simulink model "SIMULADOR_ENCODER"  (R2018a)
settings: Solver=FixedStepDiscrete  StartTime=0.0  StopTime=4  FixedStep=0.001  RelTol=1e-3
libraries: simulink x1
settings Model: Creator=Ana Araujo  LastModifiedBy=Ana Araujo

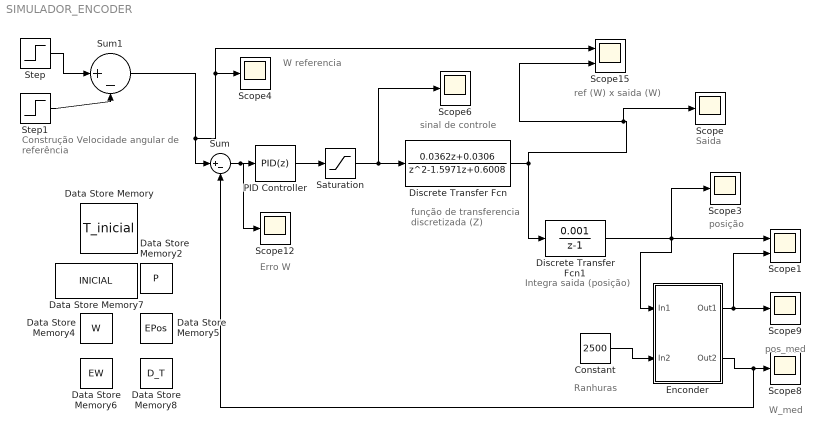
== system SIMULADOR_ENCODER ==
  note: Construção Velocidade angular
      | de referência
  note: posição
  note: Erro W
  note: Saida
  note: pos_med
  note: W_med
  note: Ranhuras
  note: função de transferencia discretizada (Z)
  note: Integra saida (posição)
  note: W referencia
  note: sinal de controle
  note: ref (W) x saida (W)
  Constant : Constant  Value=2500  SampleTime=-1
  Data Store Memory : DataStoreMemory  DataStoreName=T_inicial  ReadBeforeWriteMsg=warning  WriteAfterWriteMsg=warning  WriteAfterReadMsg=warning  ShowAdditionalParam=off
  Data Store Memory2 : DataStoreMemory  DataStoreName=P  ReadBeforeWriteMsg=warning  WriteAfterWriteMsg=warning  WriteAfterReadMsg=warning  ShowAdditionalParam=off
  Data Store Memory4 : DataStoreMemory  DataStoreName=W  ReadBeforeWriteMsg=warning  WriteAfterWriteMsg=warning  WriteAfterReadMsg=warning  ShowAdditionalParam=off
  Data Store Memory5 : DataStoreMemory  DataStoreName=EPos  ReadBeforeWriteMsg=warning  WriteAfterWriteMsg=warning  WriteAfterReadMsg=warning  ShowAdditionalParam=off
  Data Store Memory6 : DataStoreMemory  DataStoreName=EW  ReadBeforeWriteMsg=warning  WriteAfterWriteMsg=warning  WriteAfterReadMsg=warning  ShowAdditionalParam=off
  Data Store Memory7 : DataStoreMemory  DataStoreName=INICIAL  ReadBeforeWriteMsg=warning  WriteAfterWriteMsg=warning  WriteAfterReadMsg=warning  ShowAdditionalParam=off
  Data Store Memory8 : DataStoreMemory  DataStoreName=D_T  ReadBeforeWriteMsg=warning  WriteAfterWriteMsg=warning  WriteAfterReadMsg=warning  ShowAdditionalParam=off
  Discrete Transfer Fcn : DiscreteTransferFcn  Numerator="[ 0    0.0362    0.0306]"  Denominator="[1.0000   -1.5971    0.6008]"
  Discrete Transfer Fcn1 : DiscreteTransferFcn  Numerator="[ 0    0.001]"  Denominator=[ 1 -1]
  Enconder : Subsystem
  PID Controller : simulink/Continuous/PID Controller  Controller=PID  TimeDomain=Discrete-time  SampleTime=-1  IntegratorMethod=Forward Euler  FilterMethod=Forward Euler  Form=Ideal  UseFilter=off  ControllerParametersSource=internal  P=0.5  I=20  D=0.0036402852007443  N=2000  InitialConditionSource=internal  InitialConditionForIntegrator=0  InitialConditionForFilter=0  ExternalReset=none  LimitOutput=off  UpperSaturationLimit=inf  LowerSaturationLimit=-inf  LinearizeAsGain=on  AntiWindupMode=none  Kb=1  TrackingMode=off  Kt=1  PParamMin=[]  PParamMax=[]  IParamMin=[]  IParamMax=[]  DParamMin=[]  DParamMax=[]  NParamMin=[]  NParamMax=[]  KbParamMin=[]  KbParamMax=[]  KtParamMin=[]  KtParamMax=[]  POutMin=[]  POutMax=[]  IOutMin=[]  IOutMax=[]  DOutMin=[]  DOutMax=[]  NOutMin=[]  NOutMax=[]  KbOutMin=[]  KbOutMax=[]  KtOutMin=[]  KtOutMax=[]  IntegratorOutMin=[]  IntegratorOutMax=[]  FilterOutMin=[]  FilterOutMax=[]  SumOutMin=[]  SumOutMax=[]  SumI1OutMin=[]  SumI1OutMax=[]  SumI2OutMin=[]  SumI2OutMax=[]  SumI3OutMin=[]  SumI3OutMax=[]  SumDOutMin=[]  SumDOutMax=[]  SaturationOutMin=[]  SaturationOutMax=[]  IntegratorContinuousStateAttributes=''  IntegratorStateMustResolveToSignalObject=off  IntegratorRTWStateStorageClass=Auto  FilterContinuousStateAttributes=''  FilterStateMustResolveToSignalObject=off  FilterRTWStateStorageClass=Auto  DifferentiatorICPrevScaledInput=0  DifferentiatorOutMin=[]  DifferentiatorOutMax=[]  FilterDiffOutCoefMin=[]  FilterDiffOutCoefMax=[]  SumDenOutMin=[]  SumDenOutMax=[]  SumNumOutMin=[]  SumNumOutMax=[]  ReciprocalOutMin=[]  ReciprocalOutMax=[]  DivideOutMin=[]  DivideOutMax=[]  TunerSelectOption=Transfer Function Based (PID Tuner App)
  Saturation : Saturate  UpperLimit=30  LowerLimit=-30
  Scope{,3..4,6,8..9,12} (7 alike) : Scope
  Scope1 : Scope  NumInputPorts=2
  Scope15 : Scope  NumInputPorts=2
  Step : Step  Time=0  After=120  SampleTime=0
  Step1 : Step  Time=2  After=240  SampleTime=0
  Sum : Sum  Inputs=|+-
  Sum1 : Sum  Inputs=|+-
  wires:
  Discrete Transfer Fcn/1 -> Scope/1, Scope15/2, Discrete Transfer Fcn1/1
  Discrete Transfer Fcn1/1 -> Enconder/1(In1), Scope1/1, Scope3/1
  Saturation/1 -> Discrete Transfer Fcn/1, Scope6/1
  Sum/1 -> Scope12/1, PID Controller/1
  Enconder/1(Out1) -> Scope9/1, Scope1/2
  Constant/1 -> Enconder/2(In2)
  Enconder/2(Out2) -> Sum/2, Scope8/1
  PID Controller/1 -> Saturation/1
  Step/1 -> Sum1/1
  Step1/1 -> Sum1/2
  Sum1/1 -> Scope15/1, Scope4/1, Sum/1

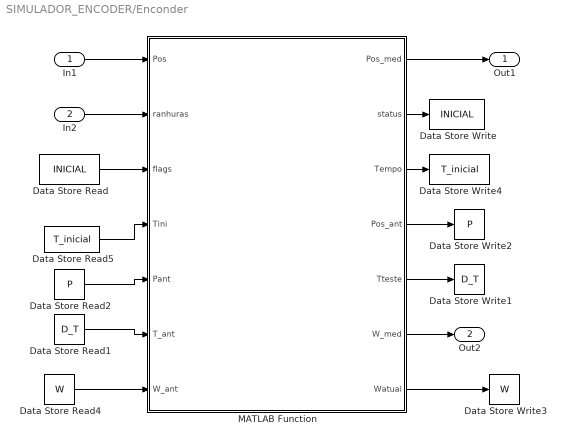
== system SIMULADOR_ENCODER/Enconder ==
  In1 : Inport
  In2 : Inport  Port=2
  Data Store Read : DataStoreRead  DataStoreName=INICIAL
  Data Store Read1 : DataStoreRead  DataStoreName=D_T
  Data Store Read2 : DataStoreRead  DataStoreName=P
  Data Store Read4 : DataStoreRead  DataStoreName=W
  Data Store Read5 : DataStoreRead  DataStoreName=T_inicial
  Data Store Write : DataStoreWrite  DataStoreName=INICIAL
  Data Store Write1 : DataStoreWrite  DataStoreName=D_T
  Data Store Write2 : DataStoreWrite  DataStoreName=P
  Data Store Write3 : DataStoreWrite  DataStoreName=W
  Data Store Write4 : DataStoreWrite  DataStoreName=T_inicial
  MATLAB Function : MATLAB Function  TreatAsAtomicUnit=on
  Out1 : Outport
  Out2 : Outport  Port=2
  wires:
  Data Store Read1/1 -> MATLAB Function/6(T_ant)
  MATLAB Function/7(Watual) -> Data Store Write3/1
  In2/1 -> MATLAB Function/2(ranhuras)
  MATLAB Function/3(Tempo) -> Data Store Write4/1
  Data Store Read5/1 -> MATLAB Function/4(Tini)
  MATLAB Function/1(Pos_med) -> Out1/1
  Data Store Read/1 -> MATLAB Function/3(flags)
  Data Store Read2/1 -> MATLAB Function/5(Pant)
  MATLAB Function/2(status) -> Data Store Write/1
  MATLAB Function/5(Tteste) -> Data Store Write1/1
  MATLAB Function/6(W_med) -> Out2/1
  MATLAB Function/4(Pos_ant) -> Data Store Write2/1
  Data Store Read4/1 -> MATLAB Function/7(W_ant)
  In1/1 -> MATLAB Function/1(Pos)

== matlab function SIMULADOR_ENCODER/Enconder/MATLAB Function ==
  data: Pos input; ranhuras input; Pos_med output; flags input; status output; Tempo output; Tini input; Pant input; Pos_ant output; Tteste output; T_ant input; W_med output; W_ant input; Watual output
function [Pos_med,status,Tempo,Pos_ant,Tteste,W_med,Watual]= ENCODER(Pos,ranhuras,flags,Tini, Pant, T_ant,W_ant)
%define dt
 dt = 0.001;
 temp = 0;
 Pos_ant = 0;

if flags == 0 %inicializa variaves:
    Pos_med = 0;
    temp = Tini;
    Pos_ant = Pos_med;
    T0=0;
    Waux=0; 
else 
    reso_ang = 2*pi/(2* ranhuras);%calcula a resolução linear
    pulsos = fix(Pos/reso_ang);%Calcula pulsos
    Pos_med= pulsos*reso_ang;
    temp = Tini + dt;
    
    if Pant~=Pos_med
        Pos_ant = Pos_med;
        T0=temp;
        Waux = (Pos_med-Pant)/(T0-T_ant);
    else
        Pos_ant=Pant;
        T0=T_ant;
        Waux = W_ant;
    end
    
end

    flags = 1;
    status = flags;
    Tempo = temp;
    Tteste=T0;
    W_med=Waux;
    Watual=W_med;
end
